simulink model "AccTarSel"  (R2018b)
settings: Solver=FixedStepDiscrete  StartTime=0.0  StopTime=inf  FixedStep=0.01  RelTol=1e-3
PostLoadFcn:
  | if any(exist('dsrtsu_mdlpostloadfcn', 'file') ~= 0), dsrtsu_mdlpostloadfcn('Execute', bdroot); end
values from neighbouring files (symbols this model uses):
  P_adtMaxBDC = 1.0    [AccTarSel.sldd]
  P_aFOCApproachIntpAcitve = -0.6    [AccTarSel.sldd]
  P_aFOCApproachIntpEnsure = -1.8    [AccTarSel.sldd]
  P_CutInEnable = 1.0    [AccTarSel.sldd]
  P_dAimMin = 4.5    [AccTarSel.sldd]
  P_dAimMinAVP = 1.5    [AccTarSel.sldd]
  P_dObjDrvOffMax = 5.0    [AccTarSel.sldd]
  P_dObjDrvOffMin = 3.0    [AccTarSel.sldd]
  P_dObjLowHystDecToStop = 4.5    [AccTarSel.sldd]
  P_dObjLowHystDecToStopAVP = 1.5    [AccTarSel.sldd]
  P_dObjUpperHystDecToStop = 5.0    [AccTarSel.sldd]
  P_dResMax = 5.0    [AccTarSel.sldd]
  P_dStandStill = 3.0    [AccTarSel.sldd]
  P_dStandStillMin = 2.0    [AccTarSel.sldd]
  P_dvarYMax4PO = 1.0    [AccTarSel.sldd]
  P_dyCutInThres = 3.6    [AccTarSel.sldd]
  P_facBDCInit = 0.7    [AccTarSel.sldd]
  P_facBDCIterCalc = 0.8    [AccTarSel.sldd]
  P_facFOCNegDiff = 0.3    [AccTarSel.sldd]
  P_facFOCPosDiff = 0.2    [AccTarSel.sldd]
  P_kapHystThres = 0.0005    [AccTarSel.sldd]
  P_PlausIntegDisable = 0.0    [AccTarSel.sldd]
  P_plausMin4PO = 0.5    [AccTarSel.sldd]
  P_probExistMin4PO = 0.8    [AccTarSel.sldd]
  P_StandObjEnable = 0.0    [AccTarSel.sldd]
  P_tAxTrackNegLower = 0.3    [AccTarSel.sldd]
  P_tAxTrackNegUpper = 0.6    [AccTarSel.sldd]
  P_tAxTrackPosLower = 1.0    [AccTarSel.sldd]
  P_tAxTrackPosUpper = 2.0    [AccTarSel.sldd]
  P_tBDCStartFilt = 0.2    [AccTarSel.sldd]
  P_tCSC = 3.5    [AccTarSel.sldd]
  P_tCurvFilt = 0.2    [AccTarSel.sldd]
  P_tCutInFilt = 0.5    [AccTarSel.sldd]
  P_tFiltAxAbsPONegFast = 0.1    [AccTarSel.sldd]
  P_tFiltAxAbsPONegSlow = 0.4    [AccTarSel.sldd]
  P_tFiltAxAbsPOPosFast = 1.2    [AccTarSel.sldd]
  P_tFiltAxAbsPOPosSlow = 2.0    [AccTarSel.sldd]
  P_tFiltAxAbsPOStand = 2.0    [AccTarSel.sldd]
  P_tFiltDAim = 0.1    [AccTarSel.sldd]
  P_tFiltDsd = 0.1    [AccTarSel.sldd]
  P_tFiltSpdLim = 3.0    [AccTarSel.sldd]
  P_tFiltVxAxPOFast = 0.15    [AccTarSel.sldd]
  P_tFiltVxAxPOSlow = 0.25    [AccTarSel.sldd]
  P_tFOCStatAccelFast = 4.0    [AccTarSel.sldd]
  P_tFOCStatAccelSlow = 3.5    [AccTarSel.sldd]
  P_tFOCStatDecelFast = 4.0    [AccTarSel.sldd]
  P_tFOCStatDecelSlow = 3.2    [AccTarSel.sldd]
  P_tMinDrvPhase = 2.0    [AccTarSel.sldd]
  P_tPredObjLeav = 1.2    [AccTarSel.sldd]
  P_tRollingFilt = 0.5    [AccTarSel.sldd]
  P_tRollingFinFilt = 1.0    [AccTarSel.sldd]
  P_tSSCNeg = 4.5    [AccTarSel.sldd]
  P_tSSCPos = 5.5    [AccTarSel.sldd]
  P_tToStop = 5.0    [AccTarSel.sldd]
  P_tToStopInBDC = 6.0    [AccTarSel.sldd]
  P_tToStopTrig = 4.0    [AccTarSel.sldd]
  P_vEgoDecToStop = 3.0    [AccTarSel.sldd]
  P_vEgoLowBDC = 4.0    [AccTarSel.sldd]
  P_vFOCNegDiff = 4.0    [AccTarSel.sldd]
  P_vFOCPosDiff = 5.0    [AccTarSel.sldd]
  P_vFOCStationaryFast = 15.0    [AccTarSel.sldd]
  P_vFOCStationarySlow = 5.0    [AccTarSel.sldd]
  P_vObjDrvOff = 0.5    [AccTarSel.sldd]
  P_vObjLowHystDecToStop = 0.5    [AccTarSel.sldd]
  P_vObjNoStop = 1.0    [AccTarSel.sldd]
  P_vObjReCalc = 1.0    [AccTarSel.sldd]
  P_vObjStop = 0.3    [AccTarSel.sldd]
  P_vObjUpperHystDecToStop = 0.8    [AccTarSel.sldd]
  P_vStandStill = 0.3    [AccTarSel.sldd]
  P_vStandStillHyst = 0.3    [AccTarSel.sldd]
  P_vyCutInThres = 0.5    [AccTarSel.sldd]
libraries: simulink x21, LPFilter x12
(part 3 of 11)

== system AccTarSel/calcCancelFlag ==
  MainState : Inport
  SYS_Info : Inport  Port=2
  AND : Logic  AllPortsSameDT=off  OutDataTypeStr=boolean
  Constant : Constant  Value=2  OutDataTypeStr=single
  Constant1 : Constant  OutDataTypeStr=single
  Constant2 : Constant  Value=0  OutDataTypeStr=single
  If : If  NumInputs=2  IfExpression=u1 ==1  ElseIfExpressions=u2 == 1
  If Action Subsystem : Subsystem  TreatAsAtomicUnit=on
  If Action Subsystem1 : Subsystem  TreatAsAtomicUnit=on
  If Action Subsystem2 : Subsystem  TreatAsAtomicUnit=on
  Memory : Memory
  Memory1 : Memory
  Merge : Merge  Inputs=3
  Merge1 : Merge  Inputs=3
  Relational Operator : RelationalOperator  OutDataTypeStr=boolean  RndMeth=Simplest
  Relational Operator1 : RelationalOperator  Operator=<=  OutDataTypeStr=boolean  RndMeth=Simplest
  Relational Operator2 : RelationalOperator  Operator=>  OutDataTypeStr=boolean  RndMeth=Simplest
  Cancel : Outport
  wires:
  MainState/1 -> Relational Operator1/1, Memory/1
  Constant/1 -> Relational Operator/2
  Memory/1 -> Relational Operator/1
  Constant1/1 -> Relational Operator1/2
  Relational Operator/1 -> AND/1
  Relational Operator1/1 -> AND/2
  AND/1 -> If/1
  If/1 -> If Action Subsystem/Action
  If Action Subsystem/1(CancelFlag) -> Merge/1
  If Action Subsystem1/1(CancelFlag) -> Merge/2
  If Action Subsystem2/1(CancelFlag) -> Merge/3
  If Action Subsystem/2(HoldTime) -> Merge1/1
  If Action Subsystem1/2(HoldTime) -> Merge1/2
  If Action Subsystem2/2(HoldTime) -> Merge1/3
  Merge1/1 -> Memory1/1
  SYS_Info/1 -> If Action Subsystem1/1(SYS_Info)
  Memory1/1 -> Relational Operator2/1, If Action Subsystem1/2(HoldTimeK1)
  If/2 -> If Action Subsystem1/Action
  If/3 -> If Action Subsystem2/Action
  Merge/1 -> Cancel/1
  Constant2/1 -> Relational Operator2/2
  Relational Operator2/1 -> If/2

== system AccTarSel/ACC_Control/AccelBoundCtrl ==
  aAM : Inport
  LowerLimitation : Subsystem
  Max : MinMax  Function=max  Inputs=2
  Max1 : MinMax  Inputs=2
  UpperLimitation : Subsystem
  aABC : Outport
  wires:
  aAM/1 -> Max/1
  LowerLimitation/1(Out1) -> Max/2
  Max/1 -> Max1/1
  UpperLimitation/1(Out1) -> Max1/2
  Max1/1 -> aABC/1

== system AccTarSel/ACC_Control/ArbitraryMix ==
  note: 00: Invalid
      | 01:Parking In
      | 02:Parking Out
      | 03:Stop
  aSSC : Inport
  FOCInfo : Inport  Port=2
  aCSC : Inport  Port=3
  aRdCrs : Inport  Port=4
  AVP_Info : Inport  Port=5
  1-D Lookup Table : Lookup_n-D  NumberOfTableDimensions=1  LookupTableObject=''  BreakpointsForDimension1=[0,1,2,3,4,5]  BreakpointsForDimension1FirstPoint=10  BreakpointsForDimension2FirstPoint=10  BreakpointsForDimension1Spacing=12  BreakpointsForDimension2Spacing=12  IndexSearchMethod=Evenly spaced points  Table=[0,1,4,3,1,5]  InterpMethod=Flat  InternalRulePriority=Speed  RndMeth=Simplest  InputSameDT=on
  Bus Creator : BusCreator  Inputs=4
  Bus Selector : BusSelector  OutputSignals=AVP_STATE
  Constant : Constant  Value=4  OutDataTypeStr=int32
  Constant1 : Constant  Value=3  OutDataTypeStr=uint8
  OR : Logic  Operator=OR  AllPortsSameDT=off  OutDataTypeStr=boolean
  Relational Operator : RelationalOperator  Operator===  OutDataTypeStr=boolean  RndMeth=Simplest
  Subsystem : Subsystem
  To Workspace5 : ToWorkspace  VariableName=aCvArray  SaveFormat=Timeseries  SampleTime=-1
  calcAFOC : Subsystem
  aAM : Outport
  DecToStop : Outport  Port=2
  CMDType : Outport  Port=3
  wires:
  aSSC/1 -> Bus Creator/1
  aCSC/1 -> Bus Creator/3
  aRdCrs/1 -> Bus Creator/4
  FOCInfo/1 -> calcAFOC/1(FOCInfo)
  calcAFOC/1(aFOC) -> Bus Creator/2
  Subsystem/1(aMin) -> aAM/1
  Bus Creator/1 -> To Workspace5/1, Subsystem/1(aCvArray)
  Constant/1 -> Subsystem/2(numASrc)
  Subsystem/2(CMDType) -> 1-D Lookup Table/1
  1-D Lookup Table/1 -> CMDType/1
  calcAFOC/2(DecToStop) -> OR/1
  Relational Operator/1 -> OR/2
  AVP_Info/1 -> Bus Selector/1
  Bus Selector/1 -> Relational Operator/1  "<AVP_STATE>"
  Constant1/1 -> Relational Operator/2
  OR/1 -> DecToStop/1

== system AccTarSel/ACC_Control/CrossRoad ==
  egoInfo : Inport
  RoadCrossInfo : Inport  Port=2
  Add : Sum  Inputs=+-
  Add1 : Sum
  Add2 : Sum  Inputs=+-
  Bus Selector : BusSelector  OutputSignals=case_num,light_des_spd,light_dist
  Bus Selector1 : BusSelector  OutputSignals=vRef
  Constant : Constant  Value=0  OutDataTypeStr=int8
  Constant1 : Constant  Value=16  OutDataTypeStr=single
  Constant2 : Constant  Value=0.1  OutDataTypeStr=single
  Constant3 : Constant  Value=0  OutDataTypeStr=single
  Constant4 : Constant  Value=0.5  OutDataTypeStr=single
  Divide : Product  Inputs=*/
  Gain : Gain  Gain=2
  Max : MinMax  Function=max  Inputs=2
  Relational Operator : RelationalOperator  Operator===  OutDataTypeStr=boolean  RndMeth=Simplest
  Square : Math  Operator=square  SaturateOnIntegerOverflow=on
  Square1 : Math  Operator=square  SaturateOnIntegerOverflow=on
  Switch : Switch  Criteria=u2 > Threshold
  aRdCrs : Outport
  wires:
  RoadCrossInfo/1 -> Bus Selector/1
  egoInfo/1 -> Bus Selector1/1
  Bus Selector/1 -> Relational Operator/1  "<case_num>"
  Constant/1 -> Relational Operator/2
  Relational Operator/1 -> Switch/2
  Constant1/1 -> Switch/1
  Bus Selector/2 -> Square/1  "<light_des_spd>"
  Bus Selector1/1 -> Square1/1  "<vRef>"
  Square/1 -> Add/1
  Square1/1 -> Add/2
  Add/1 -> Divide/1
  Gain/1 -> Add1/1
  Constant2/1 -> Add1/2
  Max/1 -> Gain/1
  Constant3/1 -> Max/2
  Add1/1 -> Divide/2
  Divide/1 -> Switch/3
  Switch/1 -> aRdCrs/1
  Bus Selector/3 -> Add2/1  "<light_dist>"
  Constant4/1 -> Add2/2
  Add2/1 -> Max/1

== system AccTarSel/ACC_Control/CurvSpdCtrl ==
  egoInfo : Inport
  EgoTraj : Inport  Port=2
  1-D Lookup Table : Lookup_n-D  NumberOfTableDimensions=1  LookupTableObject=''  BreakpointsForDimension1=[3,10,20,30]  BreakpointsForDimension1FirstPoint=10  BreakpointsForDimension2FirstPoint=10  BreakpointsForDimension1Spacing=12  BreakpointsForDimension2Spacing=12  IndexSearchMethod=Linear search  Table=[1.6,1.4,1.2,0.9]  ExtrapMethod=Clip  InternalRulePriority=Speed  RndMeth=Simplest  InputSameDT=on
  Abs : Abs
  Abs1 : Abs
  Add : Sum  Inputs=+-
  Bus Selector : BusSelector  OutputSignals=vRef,Curvature
  Constant1 : Constant  Value=0.0001  OutDataTypeStr=single
  Divide : Product  Inputs=*/
  Divide1 : Product  Inputs=*/
  Max : MinMax  Function=max  Inputs=2
  P_tSSCPos : Constant  Value=P_tCSC
  Sqrt : Sqrt  SaturateOnIntegerOverflow=on
  Terminator : Terminator
  aCSC : Outport
  wires:
  Divide1/1 -> aCSC/1
  egoInfo/1 -> Bus Selector/1
  EgoTraj/1 -> Terminator/1
  Bus Selector/1 -> Add/2, 1-D Lookup Table/1  "<vRef>"
  1-D Lookup Table/1 -> Abs1/1
  Max/1 -> Divide/2
  Bus Selector/2 -> Abs/1  "<Curvature>"
  Abs/1 -> Max/1
  Constant1/1 -> Max/2
  Divide/1 -> Sqrt/1
  Abs1/1 -> Divide/1
  Add/1 -> Divide1/1
  P_tSSCPos/1 -> Divide1/2
  Sqrt/1 -> Add/1

== system AccTarSel/ACC_Control/FollowObjCtrl ==
  StateMachine : Inport
  numFOC : Inport  Port=2
  egoInfo : Inport  Port=3
  TargetInfo : Inport  Port=4
  SYS_Info_st : Inport  Port=5
  aCvK1 : Inport  Port=6
  tTimeGapSet : Inport  Port=7
  FOCInfoK1 : Inport  Port=8
  Assignment1 : Assignment  IndexMode=Zero-based  DiagnosticForDimensions=Warning  IndexOptions=Index vector (port)  Indices=1  OutputSizes=1
  Bus Creator : BusCreator  Inputs=12  OutDataTypeStr=Bus: ACC_FOC_INFO_ST  NonVirtualBus=on
      settings: InheritFromInputs=off
  Bus Selector : BusSelector  OutputSignals=Valid
  FollowObjInvalid : Subsystem
  FollowObjValid : Subsystem
  For Iterator : ForIterator  IterationSource=external  IterationLimit=2  IndexMode=Zero-based
  If : If  IfExpression=u1 == 1
  Merge{,1..10} (11 alike) : Merge
  Selector1 : Selector  IndexMode=Zero-based  InputPortWidth=6  IndexOptions=Index vector (port)  Indices=[1 3]  OutputSizes=1
  Selector2 : Selector  IndexMode=Zero-based  InputPortWidth=6  IndexOptions=Index vector (port)  Indices=[1 3]  OutputSizes=1
  Zero1 : Constant  Value=zeros(1,6)  OutDataTypeStr=Bus: ACC_FOC_INFO_ST
  FOCInfo : Outport
  wires:
  Selector1/1 -> Bus Selector/1, FollowObjValid/3(ATS_Po_st)  "ATS_Po_st"
  Bus Selector/1 -> Bus Creator/1, If/1  "<Valid>"
  Merge/1 -> Bus Creator/2  "aFOC"
  egoInfo/1 -> FollowObjValid/2(VSI_VehState_st)
  If/1 -> FollowObjValid/Action
  If/2 -> FollowObjInvalid/Action
  FollowObjValid/1(a) -> Merge/1
  FollowObjInvalid/1(a) -> Merge/2
  FollowObjValid/2(DecToStop) -> Merge1/1
  FollowObjInvalid/2(DecToStop) -> Merge1/2
  Merge1/1 -> Bus Creator/3  "DecToStop"
  SYS_Info_st/1 -> FollowObjValid/4(SYS_Info_st)
  aCvK1/1 -> FollowObjValid/6(aCvK1)
  FollowObjInvalid/3(FirstCyc) -> Merge2/2
  FollowObjValid/3(FirstCyc) -> Merge2/1
  Merge2/1 -> Bus Creator/4  "FirstCyc"
  tTimeGapSet/1 -> FollowObjValid/7(tTimeGapSet)
  numFOC/1 -> For Iterator/1
  TargetInfo/1 -> Selector1/1  "ATS_Po_st"
  For Iterator/1 -> [i_cnt], Selector2/2, Selector1/2  "i_cnt"
  Assignment1/1 -> FOCInfo/1
  [i_cnt] -> Assignment1/3
  Zero1/1 -> Assignment1/1
  Bus Creator/1 -> Assignment1/2
  FOCInfoK1/1 -> Selector2/1
  Selector2/1 -> FollowObjValid/5(FOCInfoK1)
  FollowObjValid/4(dAim) -> Merge3/1
  FollowObjInvalid/4(dAim) -> Merge3/2
  FollowObjValid/5(aStat) -> Merge4/1
  FollowObjInvalid/5(aStat) -> Merge4/2
  FollowObjValid/6(aApproach) -> Merge5/1
  FollowObjInvalid/6(aApproach) -> Merge5/2
  FollowObjValid/7(ApproachCase) -> Merge6/1
  FollowObjInvalid/7(ApproachCase) -> Merge6/2
  FollowObjValid/8(tObjStop) -> Merge7/1
  FollowObjInvalid/8(tObjStop) -> Merge7/2
  FollowObjValid/9(dSlowDown) -> Merge8/1
  FollowObjInvalid/9(dSlowDown) -> Merge8/2
  FollowObjValid/10(ObjLeaving) -> Merge9/1
  FollowObjInvalid/10(ObjLeaving) -> Merge9/2
  Merge3/1 -> Bus Creator/5  "dAim"
  Merge4/1 -> Bus Creator/6  "aStat"
  Merge5/1 -> Bus Creator/7  "aApproach"
  Merge6/1 -> Bus Creator/8  "ApproachCase"
  Merge7/1 -> Bus Creator/9  "tObjStop"
  Merge8/1 -> Bus Creator/10  "dSlowDown"
  Merge9/1 -> Bus Creator/11  "ObjLeaving"
  StateMachine/1 -> FollowObjValid/1(StateMachine)
  FollowObjValid/11(dImmerseAdj) -> Merge10/1
  FollowObjInvalid/11(dImmerseAdj) -> Merge10/2
  Merge10/1 -> Bus Creator/12  "dImmerseAdj"

== system AccTarSel/ACC_Control/OvertakeSuppression ==
  AdjacentLaneObjInfo : Inport
  ObjList : Inport  Port=2
  egoInfo : Inport  Port=3
  AST_Info_st : Inport  Port=4
  Add : Sum
  Add1 : Sum  Inputs=+-
  Bus Selector : BusSelector  OutputSignals=L_NEIGHBORLANE_TAROBJ_2_ST.Index_un8,R_NEIGHBORLANE_TAROBJ_2_ST.Index_un8
  Bus Selector1 : BusSelector  OutputSignals=vSet
  Constant : Constant  Value=10  OutDataTypeStr=single
  Gain : Gain  Gain=1/3.6
  If : If  IfExpression=u1 <40
  If Action Subsystem : Subsystem  TreatAsAtomicUnit=on
  If Action Subsystem1 : Subsystem  TreatAsAtomicUnit=on
  If Action Subsystem2 : Subsystem  TreatAsAtomicUnit=on
  If Action Subsystem3 : Subsystem  TreatAsAtomicUnit=on
  If1 : If  IfExpression=u1 <40
  Max : MinMax  Function=max  Inputs=2
  Merge : Merge
  Merge1 : Merge
  Min : MinMax  Inputs=2
  vOvrSups : Outport
  wires:
  AdjacentLaneObjInfo/1 -> Bus Selector/1
  ObjList/1 -> If Action Subsystem2/2(TargetInfo), If Action Subsystem/2(TargetInfo)
  Bus Selector/1 -> If Action Subsystem/1(index), If/1  "<Index_un8>"
  If/1 -> If Action Subsystem/Action
  If/2 -> If Action Subsystem1/Action
  Bus Selector/2 -> If Action Subsystem2/1(index), If1/1  "<Index_un8>"
  If1/1 -> If Action Subsystem2/Action
  egoInfo/1 -> If Action Subsystem2/3(egoInfo), If Action Subsystem/3(egoInfo)
  If1/2 -> If Action Subsystem3/Action
  If Action Subsystem/1(Out1) -> Merge/1
  If Action Subsystem1/1(Out1) -> Merge/2
  If Action Subsystem2/1(Out1) -> Merge1/1
  If Action Subsystem3/1(Out1) -> Merge1/2
  Merge/1 -> Min/1
  Merge1/1 -> Min/2
  Min/1 -> Add/1
  Constant/1 -> Gain/1
  Gain/1 -> Add1/2, Add/2
  AST_Info_st/1 -> Bus Selector1/1
  Bus Selector1/1 -> Add1/1  "<vSet>"
  Add/1 -> Max/1
  Add1/1 -> Max/2
  Max/1 -> vOvrSups/1

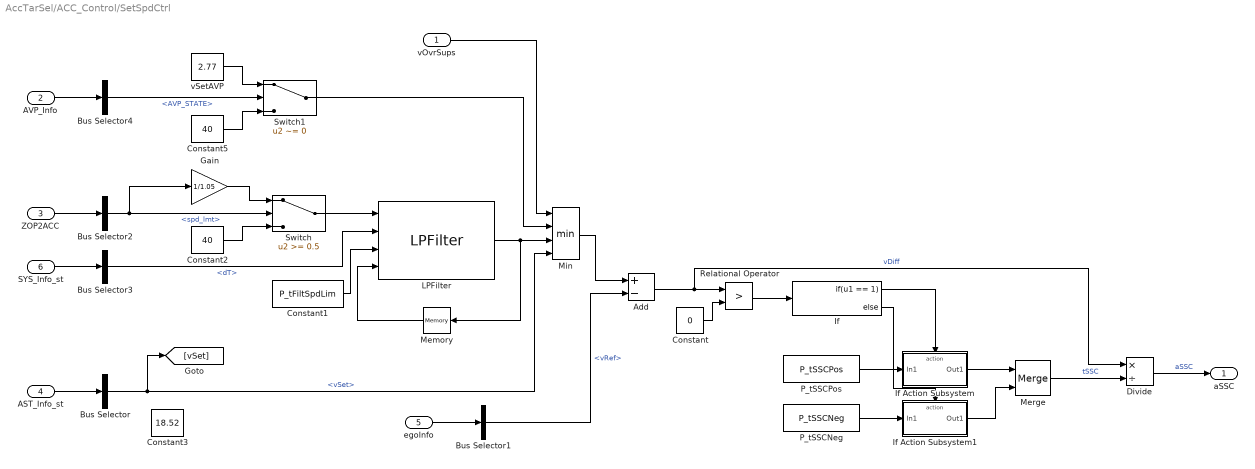
== system AccTarSel/ACC_Control/SetSpdCtrl ==
  vOvrSups : Inport
  AVP_Info : Inport  Port=2
  ZOP2ACC : Inport  Port=3
  AST_Info_st : Inport  Port=4
  egoInfo : Inport  Port=5
  SYS_Info_st : Inport  Port=6
  Add : Sum  Inputs=+-
  Bus Selector : BusSelector  OutputSignals=vSet
  Bus Selector1 : BusSelector  OutputSignals=vRef
  Bus Selector2 : BusSelector  OutputSignals=spd_lmt
  Bus Selector3 : BusSelector  OutputSignals=dT
  Bus Selector4 : BusSelector  OutputSignals=AVP_STATE
  Constant : Constant  Value=0  OutDataTypeStr=single
  Constant1 : Constant  Value=P_tFiltSpdLim
  Constant2 : Constant  Value=40  OutDataTypeStr=single
  Constant3 : Constant  Value=18.52  OutDataTypeStr=single
  Constant5 : Constant  Value=40  OutDataTypeStr=single
  Divide : Product  Inputs=*/
  Gain : Gain  Gain=1/1.05
  If : If  IfExpression=u1 == 1
  If Action Subsystem : Subsystem  TreatAsAtomicUnit=on
  If Action Subsystem1 : Subsystem  TreatAsAtomicUnit=on
  LPFilter : LPFilter/LPFilter  SystemSampleTime=-1
      settings: SourceProductName=CustomLib
  Memory : Memory  InitialCondition=40
  Merge : Merge
  Min : MinMax  Inputs=4
  P_tSSCNeg : Constant  Value=P_tSSCNeg
  P_tSSCPos : Constant  Value=P_tSSCPos
  Relational Operator : RelationalOperator  Operator=>  OutDataTypeStr=boolean  RndMeth=Simplest
  Switch : Switch  Threshold=0.5
  Switch1 : Switch  Criteria=u2 ~= 0  Threshold=0.5
  vSetAVP : Constant  Value=2.77  OutDataTypeStr=single
  aSSC : Outport
  wires:
  AST_Info_st/1 -> Bus Selector/1
  egoInfo/1 -> Bus Selector1/1
  Bus Selector1/1 -> Add/2  "<vRef>"
  Add/1 -> Divide/1, Relational Operator/1  "vDiff"
  Constant/1 -> Relational Operator/2
  Relational Operator/1 -> If/1
  P_tSSCNeg/1 -> If Action Subsystem1/1(In1)
  P_tSSCPos/1 -> If Action Subsystem/1(In1)
  If/2 -> If Action Subsystem1/Action
  If/1 -> If Action Subsystem/Action
  If Action Subsystem/1(Out1) -> Merge/1
  If Action Subsystem1/1(Out1) -> Merge/2
  Merge/1 -> Divide/2  "tSSC"
  Divide/1 -> aSSC/1  "aSSC"
  ZOP2ACC/1 -> Bus Selector2/1
  Bus Selector/1 -> [vSet], Min/4  "<vSet>"
  Min/1 -> Add/1
  Bus Selector2/1 -> Gain/1, Switch/2  "<spd_lmt>"
  Gain/1 -> Switch/1
  Switch/1 -> LPFilter/1
  SYS_Info_st/1 -> Bus Selector3/1
  Bus Selector3/1 -> LPFilter/2  "<dT>"
  Constant1/1 -> LPFilter/3
  LPFilter/1 -> Min/3, Memory/1
  Memory/1 -> LPFilter/4
  Constant2/1 -> Switch/3
  AVP_Info/1 -> Bus Selector4/1
  Bus Selector4/1 -> Switch1/2  "<AVP_STATE>"
  vSetAVP/1 -> Switch1/1
  Constant5/1 -> Switch1/3
  Switch1/1 -> Min/2
  vOvrSups/1 -> Min/1

== system AccTarSel/ACC_Target_Selection/Subsystem ==
  objInfo : Inport
  egoTrajLane_st : Inport  Port=2
  VSI_VehState_st : Inport  Port=3
  ATS_Internal_K1 : Inport  Port=4
  SYS_Info_st : Inport  Port=5
  ValidObjCalc : Subsystem  TreatAsAtomicUnit=on
  isTargetValid : Outport
  "ats_objInfo " : Outport  Port=2
  wires:
  ValidObjCalc/2("ats_objInfo ") -> "ats_objInfo "/1
  objInfo/1 -> ValidObjCalc/1(objInfo)
  egoTrajLane_st/1 -> ValidObjCalc/2(In2)
  ValidObjCalc/1(isTargetValid) -> isTargetValid/1
  VSI_VehState_st/1 -> ValidObjCalc/3(In3)
  ATS_Internal_K1/1 -> ValidObjCalc/4(ATS_Internal_K1)
  SYS_Info_st/1 -> ValidObjCalc/5(SYS_Info_st)

== system AccTarSel/ACC_Target_Selection/TargetSel ==
  isTargetValid : Inport
  objInfo : Inport  Port=2
  index : Inport  Port=3
  egoInfo : Inport  Port=4
  AND : Logic  AllPortsSameDT=off  OutDataTypeStr=boolean
  AND1 : Logic  Operator=OR  AllPortsSameDT=off  OutDataTypeStr=boolean
  Add : Sum
  Add1 : Sum
  Bus Creator : BusCreator  Inputs=11  OutDataTypeStr=Bus: ATS_PO_ST  NonVirtualBus=on
      settings: InheritFromInputs=off
  Bus Selector : BusSelector  OutputSignals=dx
  Bus Selector1 : BusSelector  OutputSignals=vRef,aRef
  Constant : Constant  Value=0  OutDataTypeStr=int32
  Constant1 : Constant  Value=0  OutDataTypeStr=boolean
  Data Type Conversion : DataTypeConversion  OutDataTypeStr=single
  Delay : Delay  DelayLength=1  InitialCondition=65535  ExternalReset=Level hold
      settings: InputPortMap=u0,r5
  Delay1 : Delay  DelayLength=1  InitialCondition=0
  If Action Subsystem : Subsystem  TreatAsAtomicUnit=on
  If Action Subsystem1 : Subsystem  TreatAsAtomicUnit=on
  If1 : If  NumInputs=2  IfExpression=u1 == 1  ElseIfExpressions=u2 == 1  ShowElse=off
  Merge{,1..8} (9 alike) : Merge
  Relational Operator : RelationalOperator  Operator=<  OutDataTypeStr=boolean  RndMeth=Simplest
  Relational Operator1 : RelationalOperator  Operator===  OutDataTypeStr=boolean  RndMeth=Simplest
  Relational Operator2 : RelationalOperator  Operator===  OutDataTypeStr=boolean  RndMeth=Simplest
  Out1 : Outport  OutDataTypeStr=Bus: ATS_PO_ST
  wires:
  isTargetValid/1 -> AND/1
  objInfo/1 -> If Action Subsystem/1(In1), Bus Selector/1
  Bus Selector/1 -> Relational Operator/1  "<dx>"
  index/1 -> Relational Operator1/1, Data Type Conversion/1
  If1/1 -> If Action Subsystem/Action
  Delay/1 -> Relational Operator/2
  Relational Operator/1 -> AND/2
  AND/1 -> If1/1
  Bus Creator/1 -> Out1/1
  Data Type Conversion/1 -> If Action Subsystem/2(In2)
  Constant/1 -> Relational Operator1/2
  AND1/1 -> Delay/2, If1/2
  If1/2 -> If Action Subsystem1/Action
  If Action Subsystem/3(dx) -> Merge/1  "dx"
  If Action Subsystem/4(dy) -> Merge1/1  "dy"
  If Action Subsystem/5(vx) -> Merge2/1  "vx"
  If Action Subsystem/6(vy) -> Merge3/1  "vy"
  If Action Subsystem/7(ax) -> Merge4/1  "ax"
  If Action Subsystem/2(index) -> Merge5/1  "Index"
  If Action Subsystem/1(valid) -> Merge6/1  "Valid"
  Merge6/1 -> Delay1/1, Bus Creator/1  "Valid"
  Merge5/1 -> Bus Creator/2  "Index"
  Merge/1 -> Delay/1, Bus Creator/3  "dx"
  Merge1/1 -> Bus Creator/4  "dy"
  Merge2/1 -> Add/1, Bus Creator/5  "vx"
  Merge3/1 -> Bus Creator/6  "vy"
  Merge4/1 -> Add1/1, Bus Creator/7  "ax"
  If Action Subsystem1/1(valid) -> Merge6/2  "Valid"
  If Action Subsystem1/2(index) -> Merge5/2  "Index"
  If Action Subsystem1/3(dx) -> Merge/2  "dx"
  If Action Subsystem1/4(dy) -> Merge1/2  "dy"
  If Action Subsystem1/5(vx) -> Merge2/2  "vx"
  If Action Subsystem1/6(vy) -> Merge3/2  "vy"
  If Action Subsystem1/7(ax) -> Merge4/2  "ax"
  If Action Subsystem1/8(Type) -> Merge7/2
  If Action Subsystem/8(Type) -> Merge7/1  "Type"
  Merge7/1 -> Bus Creator/10  "Type"
  Relational Operator1/1 -> AND1/1
  Constant1/1 -> Relational Operator2/2
  Delay1/1 -> Relational Operator2/1
  Relational Operator2/1 -> AND1/2
  egoInfo/1 -> Bus Selector1/1
  Bus Selector1/1 -> Add/2  "<vRef>"
  Add/1 -> Bus Creator/8  "vxAbs"
  Add1/1 -> Bus Creator/9  "axAbs"
  Bus Selector1/2 -> Add1/2  "<aRef>"
  If Action Subsystem/9(MotionSts) -> Merge8/1
  If Action Subsystem1/9(MotionSts) -> Merge8/2
  Merge8/1 -> Bus Creator/11  "MotionSts"

== system AccTarSel/ACC_dTarSet1/If Action Subsystem ==
  In1 : Inport
  Action Port : ActionPort  ActionType=then
  Add : Sum
  Constant : Constant  OutDataTypeStr=single
  Constant1 : Constant  Value=3  OutDataTypeStr=single
  Max : MinMax  Inputs=2
  Out1 : Outport
  wires:
  In1/1 -> Add/1
  Constant/1 -> Add/2
  Max/1 -> Out1/1
  Add/1 -> Max/1
  Constant1/1 -> Max/2

== system AccTarSel/ACC_dTarSet1/If Action Subsystem1 ==
  In1 : Inport
  Action Port : ActionPort  ActionType=elseif
  Add : Sum  Inputs=+-
  Constant : Constant  OutDataTypeStr=single
  Constant1 : Constant  OutDataTypeStr=single
  Max : MinMax  Function=max  Inputs=2
  Out1 : Outport
  wires:
  In1/1 -> Add/1
  Constant/1 -> Add/2
  Add/1 -> Max/1
  Max/1 -> Out1/1
  Constant1/1 -> Max/2
